simulink model "NoLinearModel"  (R2021b)
settings: Solver=VariableStepAuto  StartTime=tStart  StopTime=tFinal  RelTol=1e-3
values from neighbouring files (symbols this model uses):
  accelerationLimit = 0.37    [ltdSimulationParameters.m]
  ageTrain = 0.85    [ltdSimulationParameters.m]
  decelerationLimit = 1.18    [ltdSimulationParameters.m]
  Ka = 0.07    [ltdSimulationParameters.m]
  m = M * 10^3 + (load * weight)    (= 58980)    [ltdSimulationParameters.m]
  M = 54.5    [ltdSimulationParameters.m]
  maxTractiveEffort = 100 * 10 ^3    (= 100000)    [ltdSimulationParameters.m]
  nP = 6    [ltdSimulationParameters.m]
  speedLimit = 55.88    [ltdSimulationParameters.m]
  theta = 4e-4    (= 0.0004)    [ltdSimulationParameters.m]
  wP = m/nP    (= 9830)    [ltdSimulationParameters.m]
  x_1 = 0    [ltdSimulationParameters.m]
  x_2 = 0    [ltdSimulationParameters.m]
undefined symbols (not defined in the file or in its folder): magnitude
settings Model: SimulationMode=rapid-accelerator  Creator=User  LastModifiedBy=User
settings SolverCC: AlgebraicLoopSolver=TrustRegion
settings DebuggingCC: SFMachineParentedDataDiag=warning

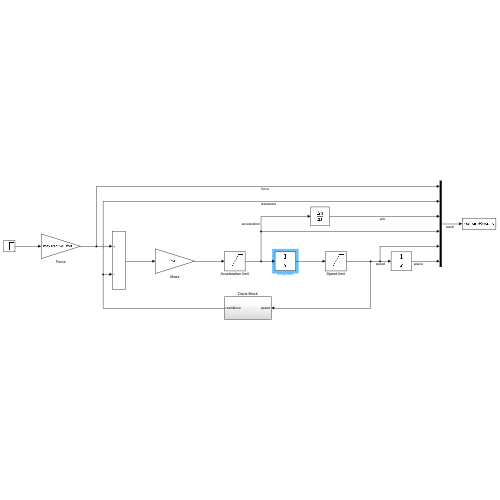
[thumbnail: Simulink's stored preview of the top-level diagram]
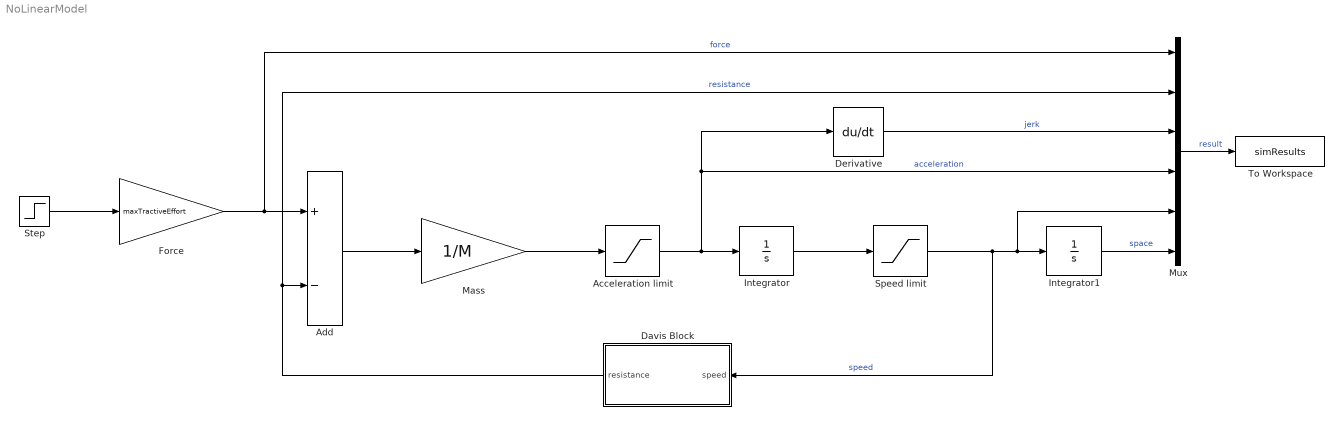
== system NoLinearModel ==
  Acceleration limit : Saturate  UpperLimit=accelerationLimit  LowerLimit=-decelerationLimit
  Add : Sum  Inputs=+-
  Davis Block : Subsystem
  Derivative : Derivative
  Force : Gain  Gain=maxTractiveEffort
  Integrator : Integrator  InitialCondition=x_2
  Integrator1 : Integrator  InitialCondition=x_1
  Mass : Gain  Gain=1/M
  Mux : Mux  Inputs=6
  Speed limit : Saturate  UpperLimit=speedLimit  LowerLimit=-speedLimit
  Step : Step  SampleTime=0
  To Workspace : ToWorkspace  VariableName=simResults  SaveFormat=Structure With Time  SampleTime=-1
  wires:
  Add/1 -> Mass/1
  Mass/1 -> Acceleration limit/1
  Acceleration limit/1 -> Derivative/1, Mux/4, Integrator/1  "acceleration"
  Integrator/1 -> Speed limit/1
  Speed limit/1 -> Davis Block/1(speed), Mux/5, Integrator1/1  "speed"
  Integrator1/1 -> Mux/6  "space"
  Derivative/1 -> Mux/3  "jerk"
  Force/1 -> Mux/1, Add/1  "force"
  Step/1 -> Force/1
  Mux/1 -> To Workspace/1  "result"
  Davis Block/1(resistance) -> Mux/2, Add/2  "resistance"

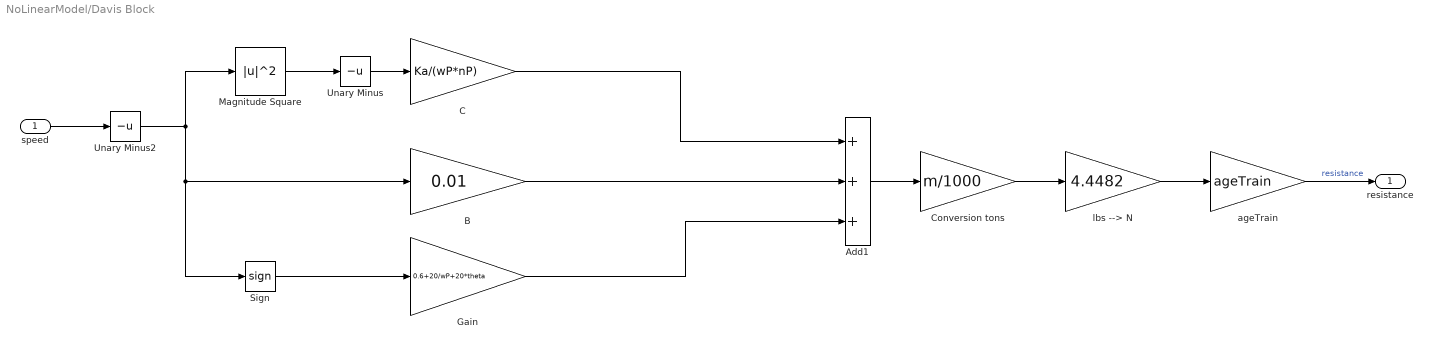
== system NoLinearModel/Davis Block ==
  speed : Inport
  Add1 : Sum  Inputs=+++
  B : Gain  Gain=0.01
  C : Gain  Gain=Ka/(wP*nP)
  Conversion tons : Gain  Gain=m/1000
  Gain : Gain  Gain=0.6+20/wP+20*theta
  Magnitude Square : Math  Operator=magnitude^2  SignedPower=on  RndMeth=Zero  SaturateOnIntegerOverflow=on
  Sign : Signum
  Unary Minus : UnaryMinus
  Unary Minus2 : UnaryMinus
  ageTrain : Gain  Gain=ageTrain
  lbs --> N : Gain  Gain=4.4482
  resistance : Outport
  wires:
  Unary Minus2/1 -> Magnitude Square/1, Sign/1, B/1
  Conversion tons/1 -> lbs --> N/1
  Add1/1 -> Conversion tons/1
  lbs --> N/1 -> ageTrain/1
  Unary Minus/1 -> C/1
  B/1 -> Add1/2
  Magnitude Square/1 -> Unary Minus/1
  Sign/1 -> Gain/1
  speed/1 -> Unary Minus2/1
  ageTrain/1 -> resistance/1  "resistance"
  C/1 -> Add1/1
  Gain/1 -> Add1/3
